simulink model "AL1adaptive"  (R2022b)
settings: Solver=ode45  StartTime=0.0  StopTime=10  RelTol=1e-6  EnableMultiTasking=on
values from neighbouring files (symbols this model uses):
  Am = (A-B*K1)    [AL1initialize.m]
  Bm = B    [AL1initialize.m]
  Bum = [     1     0     0     0     0     0     0     0;     0     1     0     0     0     0     0     0;     0     0     0     0     0     0     0     0;     0     0     0     0     0     0     0     0;     0     0     0     0     0     0     0     0;     0     0     0     0     0     0     0     0;     0     0     1     0     0     0     0     0;     0     0     0     1     0     0     0     0;     0  ...(+189 chars)    [AL1initialize.m]
  C_full = [     0 0 0     0 0 0    1 0 0    0 0 0;     0 0 0     0 0 0    0 1 0    0 0 0;     0 0 0     0 0 0    0 0 1    0 0 0;     0 0 0     0 0 0    0 0 0    1 0 0;     0 0 0     0 0 0    0 0 0    0 1 0;     0 0 0     0 0 0    0 0 0    0 0 1]    [AL1initialize.m]
  D = zeros(4,4)    [AL1initialize.m]
  Deltabound = 1    [AL1initialize.m]
  HD = ss(zeros(4,4),eye(4),eye(4),zeros(4,4))    [AL1initialize.m]
  HmHum = ss(HmHumprop)    [AL1initialize.m]
  K1 = lqr(A,B,Q,R)    [AL1initialize.m]
  K2 = eye(4)*10    [AL1initialize.m]
  Kg = -(C*Am^-1*Bm)^-1    [AL1initialize.m]
  Lambda = [ ... (first row only)    [AL1initialize.m]
  PBmG = P*Bm*Gamma    [AL1initialize.m]
  PBumG = P*Bum*Gamma    [AL1initialize.m]
  V_trim = [v_trim; v_trim; v_trim; v_trim]    [AL1initialize.m]
  vfail = (12)^(1/3.88)    (= 1.89731524545)    [AL1initialize.m]
  Vmax = 12.5    [AL1initialize.m]
  x_initial = [0;0;0;0;0;0;0;0;0;0;0;0]    [AL1initialize.m]
libraries: Projection x8, matrix_library x6, simulink_extras x4
settings Model: Creator=oldmao  LastModifiedBy=HY
settings SolverCC: AlgebraicLoopSolver=TrustRegion
settings DataIOCC: LimitDataPoints=on  SaveFormat=Array  SignalLoggingSaveFormat=ModelDataLogs  ReturnWorkspaceOutputs=off
settings OptimizationCC: ExpressionDepthLimit=2147483647  LifeSpan=inf
settings DebuggingCC: UnderspecifiedInitializationDetection=Classic  MergeDetectMultiDrivingBlocksExec=none  SolverPrmCheckMsg=warning  FcnCallInpInsideContextMsg=warning  UnconnectedInputMsg=warning  UnconnectedOutputMsg=warning  UnconnectedLineMsg=warning  AllowSymbolicDim=off  StateNameClashWarn=warning  SFUnexpectedBacktrackingDiag=warning  SFNoUnconditionalDefaultTransitionDiag=warning  SFExecutionAtInitializationDiag=none  SFMachineParentedDataDiag=warning  ArithmeticOperatorsInVariantConditions=warning
settings HardwareCC: ProdBitPerPointer=32  ProdBitPerSizeT=32  ProdBitPerPtrDiffT=32  ProdLargestAtomicFloat=None  ProdIntDivRoundTo=Undefined  ProdEndianess=Unspecified  ProdWordSize=32  ProdHWDeviceType=32-bit Generic
settings ModelReferenceCC: EnableRefExpFcnMdlSchedulingChecks=on  PropagateSignalLabelsOutOfModel=off
settings SFSimCC: SimUseLocalCustomCode=off  CustomCodeUndefinedFunction=UseInterfaceOnly
settings RTWCC: RTWUseLocalCustomCode=off
settings CodeAppCC: StateflowObjectComments=on
settings GRTTargetCC: TargetLangStandard=C89/C90 (ANSI)  CombineOutputUpdateFcns=off  GRTInterface=on
settings ConfigComp: CovMetricSettings=dw  CovSaveCumulativeToWorkspaceVar=on  CovSaveSingleToWorkspaceVar=on  CovExternalEMLEnable=off  CovSFcnEnable=off

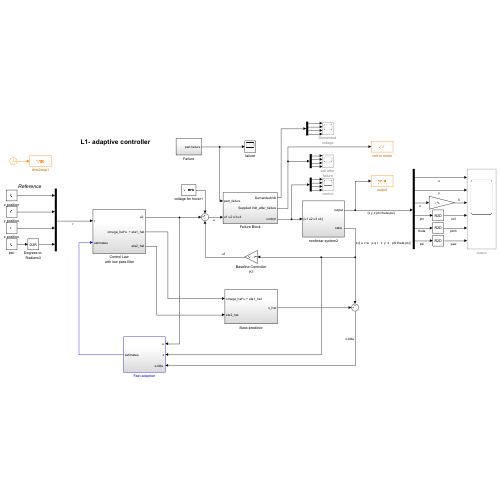
[thumbnail: Simulink's stored preview of the top-level diagram]
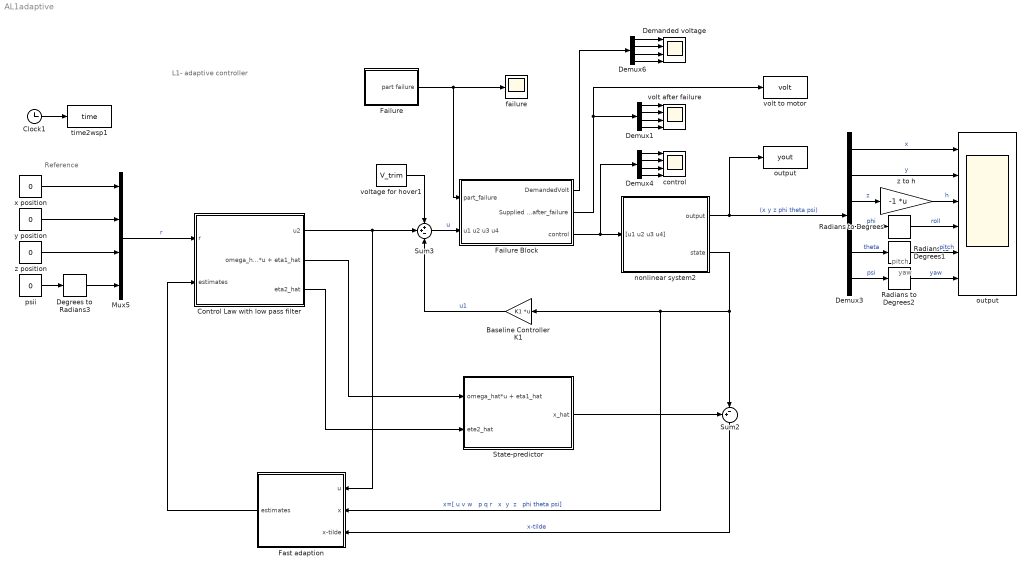
== system AL1adaptive ==
  note: Reference
  note: yaw
  note: pitch
  note: L1- adaptive controller
  Baseline Controller K1 : Gain  Gain=K1  Multiplication=Matrix(K*u) (u vector)
  Clock1 : Clock
  Control Law with low pass filter : Subsystem
  Degrees to Radians3 : simulink_extras/Transformations/Degrees to Radians
  Demanded voltage : Scope  NumInputPorts=4
  Demux1 : Demux
  Demux3 : Demux  Outputs=6
  Demux4 : Demux
  Demux6 : Demux
  Failure : Subsystem
  Failure Block : Subsystem
  Fast adaption : Subsystem
  Mux5 : Mux
  Radians to Degrees : simulink_extras/Transformations/Radians to Degrees
  Radians to Degrees1 : simulink_extras/Transformations/Radians to Degrees
  Radians to Degrees2 : simulink_extras/Transformations/Radians to Degrees
  State-predictor : Subsystem
  Sum2 : Sum  Inputs=+-|
  Sum3 : Sum  Inputs=++-
  "control " : Scope  NumInputPorts=4
  failure : Scope
  nonlinear system2 : Subsystem
  output : ToWorkspace  VariableName=yout  SaveFormat=Structure With Time  SampleTime=-1
  "output " : Scope  NumInputPorts=6
  "psii " : Constant  Value=0
  time2wsp1 : ToWorkspace  VariableName=time  SampleTime=-1
  volt after failure : Scope  NumInputPorts=4
  volt to motor : ToWorkspace  VariableName=volt  SaveFormat=Structure With Time  SampleTime=-1
  voltage for hover1 : Constant  Value=V_trim
  x position : Constant  Value=0
  "y position " : Constant  Value=0
  z position : Constant  Value=0
  z to h : Gain  Gain=-1  Multiplication=Matrix(K*u)
  wires:
  Clock1/1 -> time2wsp1/1
  Sum2/1 -> Fast adaption/3("x-tilde ")  "x-tilde"
  Sum3/1 -> Failure Block/2(u1 u2 u3 u4)  "u"
  Demux3/3 -> z to h/1  "z"
  Baseline Controller K1/1 -> Sum3/3  "u1"
  Failure Block/3(control) -> Demux4/1, nonlinear system2/1("[u1 u2 u3 u4]")
  Demux1/1 -> volt after failure/1
  Demux1/3 -> volt after failure/3
  Demux1/2 -> volt after failure/2
  Demux1/4 -> volt after failure/4
  Demux4/1 -> "control "/1
  Demux4/3 -> "control "/3
  Demux4/2 -> "control "/2
  Demux4/4 -> "control "/4
  Demux3/4 -> Radians to Degrees/1  "phi"
  Demux3/5 -> Radians to Degrees1/1  "theta"
  Demux3/6 -> Radians to Degrees2/1  "psi"
  Demux3/1 -> "output "/1  "x"
  nonlinear system2/2("state ") -> Baseline Controller K1/1, Fast adaption/2(x), Sum2/2  "x=[ u v w   p q r   x  y  z   phi theta psi]"
  "psii "/1 -> Degrees to Radians3/1
  z position/1 -> Mux5/3
  "y position "/1 -> Mux5/2
  x position/1 -> Mux5/1
  voltage for hover1/1 -> Sum3/1
  nonlinear system2/1(output) -> Demux3/1, output/1  "(x y z phi theta psi)"
  Radians to Degrees2/1 -> "output "/6  "yaw"
  Radians to Degrees1/1 -> "output "/5  "pitch"
  Radians to Degrees/1 -> "output "/4  "roll"
  z to h/1 -> "output "/3  "h"
  Demux3/2 -> "output "/2  "y"
  Failure/1(part failure) -> Failure Block/1("part_failure "), failure/1
  Demux6/1 -> Demanded voltage/1
  Demux6/3 -> Demanded voltage/3
  Demux6/2 -> Demanded voltage/2
  Demux6/4 -> Demanded voltage/4
  Failure Block/1(" DemandedVolt") -> Demux6/1
  Failure Block/2(Supplied Volt_after_failure) -> volt to motor/1, Demux1/1
  Degrees to Radians3/1 -> Mux5/4
  State-predictor/1(x_hat) -> Sum2/1
  Control Law with low pass filter/1("u2 ") -> Fast adaption/1(u), Sum3/2
  Mux5/1 -> Control Law with low pass filter/1(r)  "r"
  Fast adaption/1(estimates) -> Control Law with low pass filter/2(estimates)
  Control Law with low pass filter/2(omega_hat*u + eta1_hat) -> State-predictor/1(omega_hat*u + eta1_hat)
  Control Law with low pass filter/3(eta2_hat) -> State-predictor/2(ete2_hat)

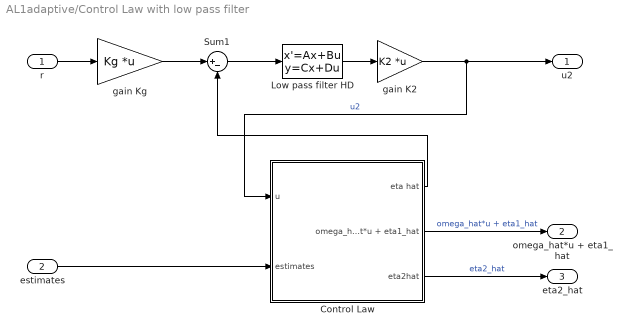
== system AL1adaptive/Control Law with low pass filter ==
  r : Inport
  estimates : Inport  Port=2
  Control Law : Subsystem
  Low pass filter HD : StateSpace  A=HD.a  B=HD.b  C=HD.c  D=HD.d  InitialCondition=0
  Sum1 : Sum  Inputs=|+-
  gain K2 : Gain  Gain=K2  Multiplication=Matrix(K*u) (u vector)
  gain Kg : Gain  Gain=Kg  Multiplication=Matrix(K*u)
  "u2 " : Outport
  omega_hat*u + eta1_hat : Outport  Port=2
  eta2_hat : Outport  Port=3
  wires:
  estimates/1 -> Control Law/2(estimates)
  Low pass filter HD/1 -> gain K2/1
  r/1 -> gain Kg/1
  Control Law/1(eta hat) -> Sum1/2
  gain K2/1 -> Control Law/1(u), "u2 "/1  "u2"
  Sum1/1 -> Low pass filter HD/1
  gain Kg/1 -> Sum1/1
  Control Law/2(omega_hat*u + eta1_hat) -> omega_hat*u + eta1_hat/1  "omega_hat*u + eta1_hat"
  Control Law/3(eta2hat) -> eta2_hat/1  "eta2_hat"

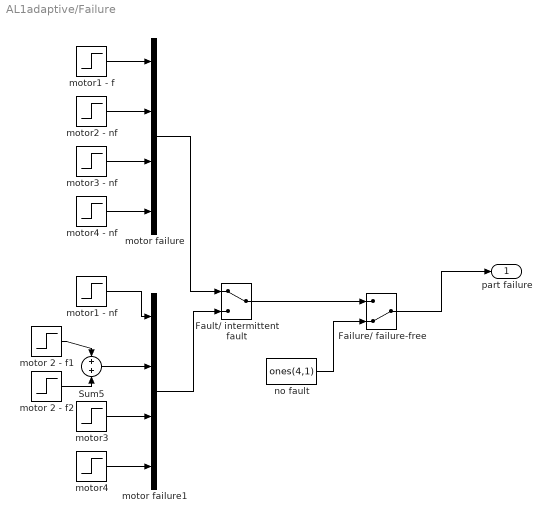
== system AL1adaptive/Failure ==
  Failure/ failure-free : ManualSwitch  CurrentSetting=0
  Fault/ intermittent fault : ManualSwitch
  Sum5 : Sum  Inputs=+|+
  motor 2 - f1 : Step  Before=1  After=0.5  SampleTime=0
  motor 2 - f2 : Step  Time=3  After=0.5  SampleTime=0
  motor failure : Concatenate  NumInputs=4
  motor failure1 : Concatenate  NumInputs=4
  motor1 - f : Step  Before=1  After=(vfail)^(3.88)  SampleTime=0
  motor1 - nf : Step  Time=5  Before=1  SampleTime=0
  motor2 - nf : Step  Before=1  SampleTime=0
  motor3 : Step  Time=5  Before=1  SampleTime=0
  motor3 - nf : Step  Time=5  Before=1  SampleTime=0
  motor4 : Step  Time=5  Before=1  SampleTime=0
  motor4 - nf : Step  Time=5  Before=1  SampleTime=0
  no fault : Constant  Value=ones(4,1)
  part failure : Outport
  wires:
  motor4/1 -> motor failure1/4
  motor3/1 -> motor failure1/3
  motor failure1/1 -> Fault/ intermittent fault/2
  motor 2 - f2/1 -> Sum5/2
  motor 2 - f1/1 -> Sum5/1
  motor4 - nf/1 -> motor failure/4
  motor3 - nf/1 -> motor failure/3
  motor2 - nf/1 -> motor failure/2
  motor1 - f/1 -> motor failure/1
  motor failure/1 -> Fault/ intermittent fault/1
  Fault/ intermittent fault/1 -> Failure/ failure-free/1
  Failure/ failure-free/1 -> part failure/1
  no fault/1 -> Failure/ failure-free/2
  motor1 - nf/1 -> motor failure1/1
  Sum5/1 -> motor failure1/2

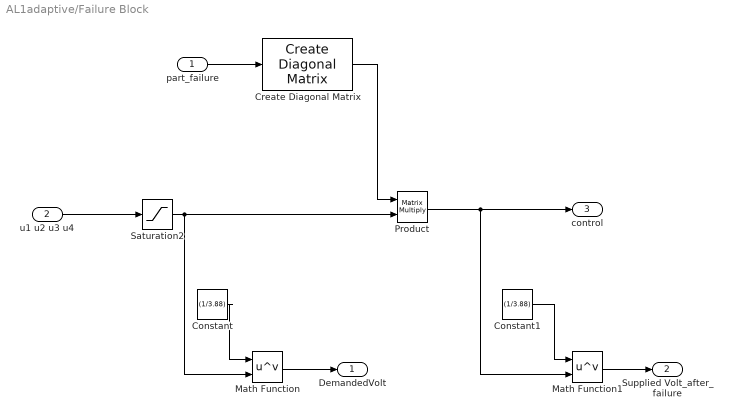
== system AL1adaptive/Failure Block ==
  "part_failure " : Inport
  u1 u2 u3 u4 : Inport  Port=2
  Constant : Constant  Value=(1/3.88)
  Constant1 : Constant  Value=(1/3.88)
  Create Diagonal Matrix : matrix_library/Create Diagonal Matrix
  Math Function : Math  Operator=pow
  Math Function1 : Math  Operator=pow
  Product : Product  Multiplication=Matrix(*)  RndMeth=Zero
  Saturation2 : Saturate  UpperLimit=Vmax^(3.88)  LowerLimit=0
  " DemandedVolt" : Outport
  Supplied Volt_after_failure : Outport  Port=2
  control : Outport  Port=3
  wires:
  Create Diagonal Matrix/1 -> Product/1
  "part_failure "/1 -> Create Diagonal Matrix/1
  Math Function/1 -> " DemandedVolt"/1
  u1 u2 u3 u4/1 -> Saturation2/1
  Saturation2/1 -> Product/2, Math Function/2
  Product/1 -> Math Function1/2, control/1
  Constant/1 -> Math Function/1
  Constant1/1 -> Math Function1/1
  Math Function1/1 -> Supplied Volt_after_failure/1

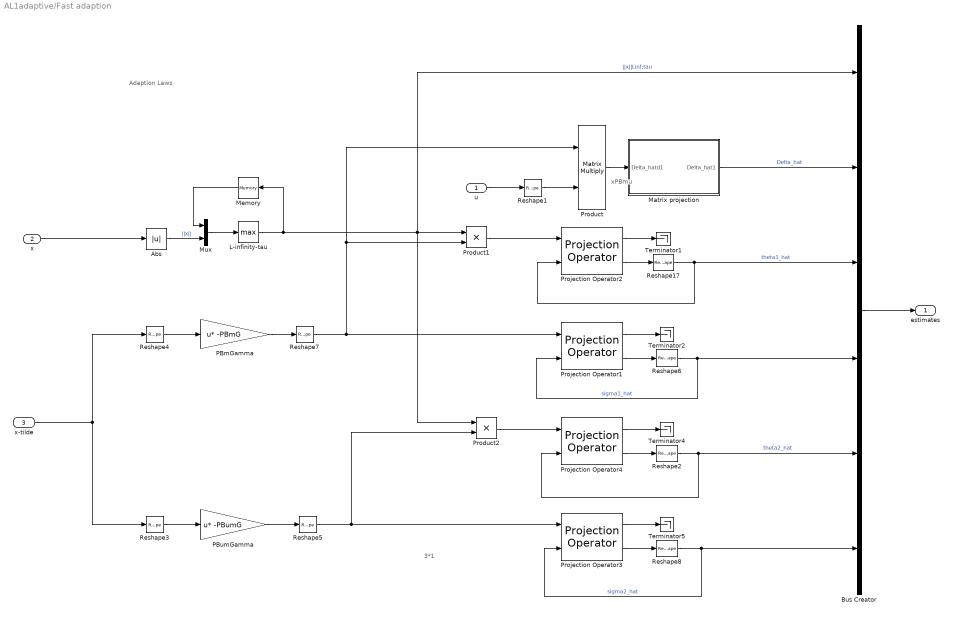
== system AL1adaptive/Fast adaption ==
  note: Adaption Laws
  note: xPBmu
  note: 3*1
  u : Inport
  x : Inport  Port=2
  "x-tilde " : Inport  Port=3
  Abs : Abs  SaturateOnIntegerOverflow=off
  Bus Creator : BusCreator  Inputs=6
  L-infinity-tau : MinMax  Function=max
  Matrix projection : Subsystem
  Memory : Memory
  Mux : Mux  Inputs=2
  PBmGamma : Gain  Gain=-PBmG  Multiplication=Matrix(u*K)
  PBumGamma : Gain  Gain=-PBumG  Multiplication=Matrix(u*K)
  Product : Product  Multiplication=Matrix(*)  RndMeth=Zero
  Product1 : Product  RndMeth=Zero
  Product2 : Product  RndMeth=Zero
  Projection Operator1 : Projection/Projection Operator  EpsilonTheta=.1  Prmax=sigama1hatbound  Prcenter=0  Pr0=0
  Projection Operator2 : Projection/Projection Operator  EpsilonTheta=.1  Prmax=theta1hatbound  Prcenter=0  Pr0=0
  Projection Operator3 : Projection/Projection Operator  EpsilonTheta=.1  Prmax=sigama2hatbound  Prcenter=0  Pr0=0
  Projection Operator4 : Projection/Projection Operator  EpsilonTheta=.1  Prmax=theta2hatbound  Prcenter=0  Pr0=0
  Reshape1 : Reshape  OutputDimensionality=Row vector (2-D)
  Reshape{2,5..8,17} (6 alike) : Reshape  OutputDimensionality=Column vector (2-D)
  Reshape3 : Reshape  OutputDimensionality=Row vector (2-D)
  Reshape4 : Reshape  OutputDimensionality=Row vector (2-D)
  Terminator{1..2,4..5} (4 alike) : Terminator
  estimates : Outport
  wires:
  x/1 -> Abs/1
  Projection Operator2/2 -> Reshape17/1
  Projection Operator2/1 -> Terminator1/1
  Reshape17/1 -> Projection Operator2/2, Bus Creator/3  "theta1_hat"
  Projection Operator1/2 -> Reshape6/1
  Projection Operator1/1 -> Terminator2/1
  u/1 -> Reshape1/1
  Reshape4/1 -> PBmGamma/1
  Reshape1/1 -> Product/2
  Product1/1 -> Projection Operator2/1
  PBmGamma/1 -> Reshape7/1
  "x-tilde "/1 -> Reshape4/1, Reshape3/1
  Reshape7/1 -> Projection Operator1/1, Product1/2, Product/1
  Projection Operator4/2 -> Reshape2/1
  Projection Operator4/1 -> Terminator4/1
  Projection Operator3/2 -> Reshape8/1
  Projection Operator3/1 -> Terminator5/1
  Reshape3/1 -> PBumGamma/1
  Product2/1 -> Projection Operator4/1
  PBumGamma/1 -> Reshape5/1
  Reshape5/1 -> Product2/2, Projection Operator3/1
  Reshape6/1 -> Projection Operator1/2, Bus Creator/4  "sigma1_hat"
  Product/1 -> Matrix projection/1(Delta_hatd1)
  Matrix projection/1(Delta_hat1) -> Bus Creator/2  "Delta_hat"
  Reshape2/1 -> Projection Operator4/2, Bus Creator/5  "theta2_hat"
  Reshape8/1 -> Projection Operator3/2, Bus Creator/6  "sigma2_hat"
  Abs/1 -> Mux/2  "||x||"
  Mux/1 -> L-infinity-tau/1
  Memory/1 -> Mux/1
  L-infinity-tau/1 -> Memory/1, Product2/1, Bus Creator/1, Product1/1  "||x||Linf;tau"
  Bus Creator/1 -> estimates/1

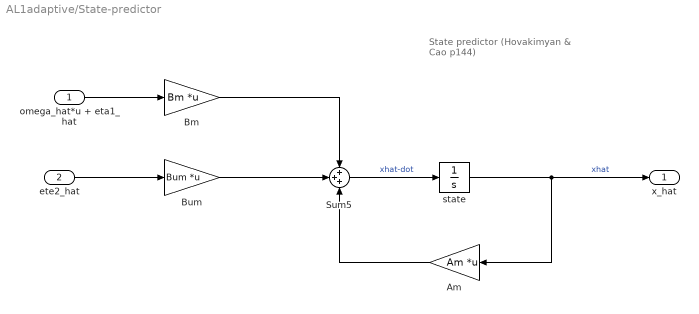
== system AL1adaptive/State-predictor ==
  note: State predictor
      | (Hovakimyan & Cao p144)
  omega_hat*u + eta1_hat : Inport
  ete2_hat : Inport  Port=2
  Am : Gain  Gain=Am  Multiplication=Matrix(K*u) (u vector)
  Bm : Gain  Gain=Bm  Multiplication=Matrix(K*u) (u vector)
  Bum : Gain  Gain=Bum  Multiplication=Matrix(K*u) (u vector)
  Sum5 : Sum  Inputs=+++
  state : Integrator  InitialCondition=x_initial
  x_hat : Outport
  wires:
  Am/1 -> Sum5/3
  Sum5/1 -> state/1  "xhat-dot"
  state/1 -> x_hat/1, Am/1  "xhat"
  ete2_hat/1 -> Bum/1
  omega_hat*u + eta1_hat/1 -> Bm/1
  Bum/1 -> Sum5/2
  Bm/1 -> Sum5/1

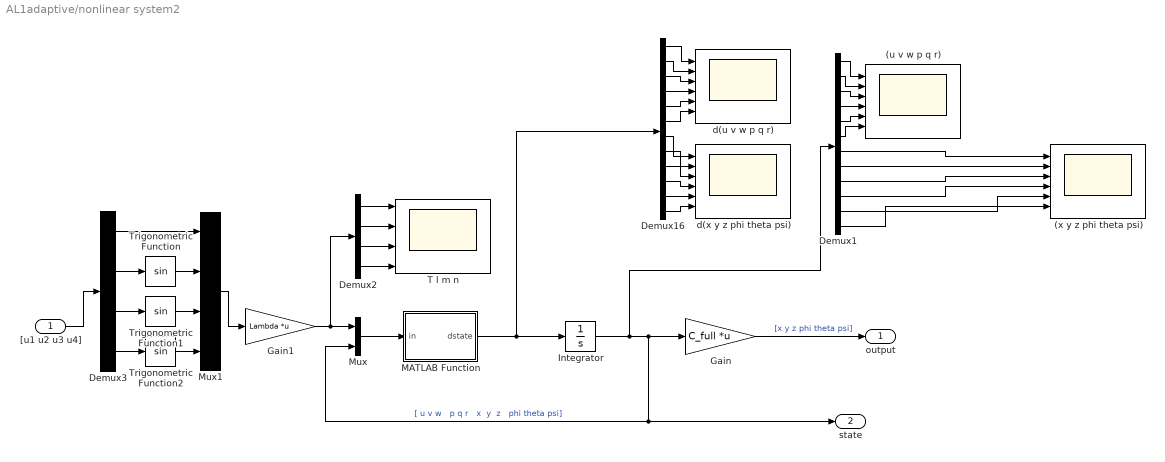
== system AL1adaptive/nonlinear system2 ==
  "[u1 u2 u3 u4]" : Inport
  (u v w p q r) : Scope  NumInputPorts=6
  (x y z phi theta psi) : Scope  NumInputPorts=6
  Demux1 : Demux  Outputs=12
  Demux16 : Demux  Outputs=12
  Demux2 : Demux
  Demux3 : Demux
  Gain : Gain  Gain=C_full  Multiplication=Matrix(K*u)
  Gain1 : Gain  Gain=Lambda  Multiplication=Matrix(K*u)
  Integrator : Integrator  InitialCondition=x_initial
  MATLAB Function : MATLAB Function  TreatAsAtomicUnit=on
  Mux : Mux  Inputs=2
  Mux1 : Mux
  T l m n : Scope  NumInputPorts=4
  Trigonometric Function : Trigonometry
  Trigonometric Function1 : Trigonometry
  Trigonometric Function2 : Trigonometry
  d(u v w p q r) : Scope  NumInputPorts=6
  d(x y z phi theta psi) : Scope  NumInputPorts=6
  output : Outport
  "state " : Outport  Port=2
  wires:
  Gain/1 -> output/1  "[x y z phi theta psi]"
  Mux/1 -> MATLAB Function/1(in)
  Integrator/1 -> Demux1/1, Gain/1, "state "/1, Mux/2  "[ u v w   p q r   x  y  z   phi theta psi]"
  Demux16/1 -> d(u v w p q r)/1
  Demux16/3 -> d(u v w p q r)/3
  Demux16/2 -> d(u v w p q r)/2
  Demux16/4 -> d(u v w p q r)/4
  Demux16/12 -> d(x y z phi theta psi)/6
  Demux16/11 -> d(x y z phi theta psi)/5
  Demux16/10 -> d(x y z phi theta psi)/4
  Demux16/9 -> d(x y z phi theta psi)/3
  Demux16/8 -> d(x y z phi theta psi)/2
  Demux16/7 -> d(x y z phi theta psi)/1
  Demux16/5 -> d(u v w p q r)/5
  Demux16/6 -> d(u v w p q r)/6
  Demux1/1 -> (u v w p q r)/1
  Demux1/3 -> (u v w p q r)/3
  Demux1/2 -> (u v w p q r)/2
  Demux1/4 -> (u v w p q r)/4
  Demux1/12 -> (x y z phi theta psi)/6
  Demux1/11 -> (x y z phi theta psi)/5
  Demux1/10 -> (x y z phi theta psi)/4
  Demux1/9 -> (x y z phi theta psi)/3
  Demux1/8 -> (x y z phi theta psi)/2
  Demux1/7 -> (x y z phi theta psi)/1
  Demux1/5 -> (u v w p q r)/5
  Demux1/6 -> (u v w p q r)/6
  Gain1/1 -> Demux2/1, Mux/1
  MATLAB Function/1(dstate) -> Demux16/1, Integrator/1
  Demux2/1 -> T l m n/1
  Demux2/2 -> T l m n/2
  Demux2/3 -> T l m n/3
  Demux2/4 -> T l m n/4
  Demux3/3 -> Trigonometric Function1/1
  Demux3/2 -> Trigonometric Function/1
  Demux3/1 -> Mux1/1
  Demux3/4 -> Trigonometric Function2/1
  "[u1 u2 u3 u4]"/1 -> Demux3/1
  Trigonometric Function1/1 -> Mux1/3
  Trigonometric Function/1 -> Mux1/2
  Trigonometric Function2/1 -> Mux1/4
  Mux1/1 -> Gain1/1

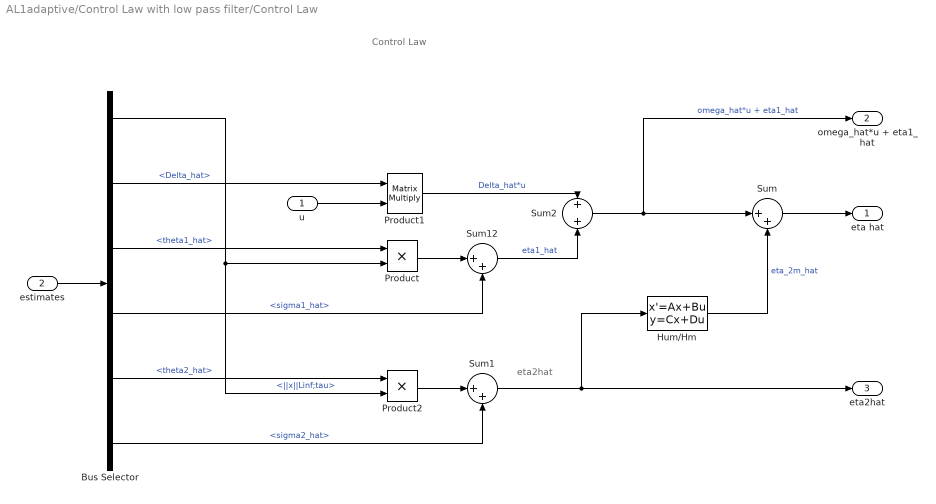
== system AL1adaptive/Control Law with low pass filter/Control Law ==
  note: Control Law
  note: eta2hat
  u : Inport
  estimates : Inport  Port=2
  Bus Selector : BusSelector  OutputSignals=||x||Linf;tau,Delta_hat,theta1_hat,sigma1_hat,theta2_hat,sigma2_hat
  "Hum/Hm " : StateSpace  A=HmHum.a  B=HmHum.b  C=HmHum.c  D=HmHum.d  InitialCondition=0
  Product : Product  RndMeth=Zero
  Product1 : Product  Multiplication=Matrix(*)  RndMeth=Zero
  Product2 : Product  RndMeth=Zero
  Sum : Sum  Inputs=|++
  Sum1 : Sum  Inputs=|++
  Sum12 : Sum  Inputs=|++
  Sum2 : Sum  Inputs=+|+
  eta hat : Outport
  omega_hat*u + eta1_hat : Outport  Port=2
  eta2hat : Outport  Port=3
  wires:
  Bus Selector/3 -> Product/1  "<theta1_hat>"
  Bus Selector/4 -> Sum12/2  "<sigma1_hat>"
  Bus Selector/5 -> Product2/1  "<theta2_hat>"
  Product2/1 -> Sum1/1
  Bus Selector/6 -> Sum1/2  "<sigma2_hat>"
  Bus Selector/2 -> Product1/1  "<Delta_hat>"
  u/1 -> Product1/2
  Sum1/1 -> "Hum/Hm "/1, eta2hat/1
  Sum/1 -> eta hat/1
  "Hum/Hm "/1 -> Sum/2  "eta_2m_hat"
  Product/1 -> Sum12/1
  Sum2/1 -> omega_hat*u + eta1_hat/1, Sum/1  "omega_hat*u + eta1_hat"
  Sum12/1 -> Sum2/2  "eta1_hat"
  Product1/1 -> Sum2/1  "Delta_hat*u"
  Bus Selector/1 -> Product2/2, Product/2  "<||x||Linf;tau>"
  estimates/1 -> Bus Selector/1

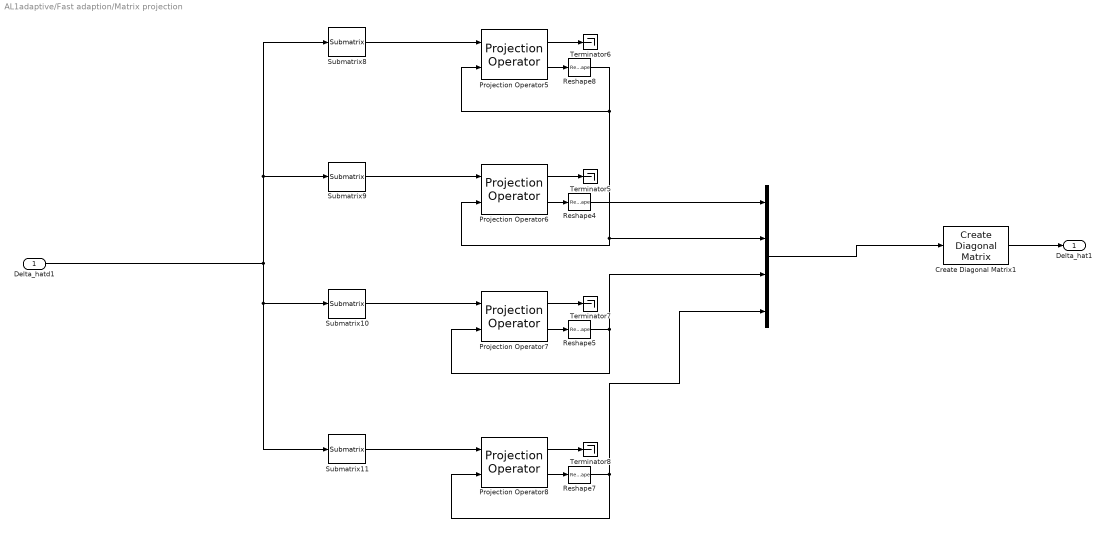
== system AL1adaptive/Fast adaption/Matrix projection ==
  Delta_hatd1 : Inport
  " " : Concatenate  NumInputs=4
  Create Diagonal Matrix1 : matrix_library/Create Diagonal Matrix
  Projection Operator5 : Projection/Projection Operator  EpsilonTheta=.1  Prmax=Deltabound/2  Prcenter=0.5  Pr0=1
  Projection Operator6 : Projection/Projection Operator  EpsilonTheta=.1  Prmax=Deltabound/2  Prcenter=0.5  Pr0=1
  Projection Operator7 : Projection/Projection Operator  EpsilonTheta=.1  Prmax=Deltabound/2  Prcenter=0.5  Pr0=1
  Projection Operator8 : Projection/Projection Operator  EpsilonTheta=0.1  Prmax=Deltabound/2  Prcenter=0.5  Pr0=1
  Reshape{4..5,7..8} (4 alike) : Reshape  OutputDimensionality=Column vector (2-D)
  Submatrix10 : matrix_library/Submatrix  RowSpan=One row  RowStartMode=Index  RowStartIndex=3  RowEndMode=Last  RowEndIndex=1  ColSpan=One column  ColStartMode=Index  ColStartIndex=3  ColEndMode=Last  ColEndIndex=1
  Submatrix11 : matrix_library/Submatrix  RowSpan=One row  RowStartMode=Index  RowStartIndex=4  RowEndMode=Last  RowEndIndex=1  ColSpan=One column  ColStartMode=Index  ColStartIndex=4  ColEndMode=Last  ColEndIndex=1
  Submatrix8 : matrix_library/Submatrix  RowSpan=One row  RowStartMode=Index  RowStartIndex=1  RowEndMode=Last  RowEndIndex=1  ColSpan=One column  ColStartMode=Index  ColStartIndex=1  ColEndMode=Last  ColEndIndex=1
  Submatrix9 : matrix_library/Submatrix  RowSpan=One row  RowStartMode=Index  RowStartIndex=2  RowEndMode=Last  RowEndIndex=1  ColSpan=One column  ColStartMode=Index  ColStartIndex=2  ColEndMode=Last  ColEndIndex=1
  Terminator{5..8} (4 alike) : Terminator
  Delta_hat1 : Outport
  wires:
  Submatrix8/1 -> Projection Operator5/1
  Projection Operator5/1 -> Terminator6/1
  Projection Operator5/2 -> Reshape8/1
  Submatrix10/1 -> Projection Operator7/1
  Projection Operator7/1 -> Terminator7/1
  Projection Operator7/2 -> Reshape5/1
  Reshape5/1 -> " "/3, Projection Operator7/2
  Reshape4/1 -> Projection Operator6/2, " "/2
  Projection Operator6/1 -> Terminator5/1
  Projection Operator6/2 -> Reshape4/1
  Create Diagonal Matrix1/1 -> Delta_hat1/1
  Submatrix9/1 -> Projection Operator6/1
  Reshape8/1 -> " "/1, Projection Operator5/2
  Submatrix11/1 -> Projection Operator8/1
  Projection Operator8/1 -> Terminator8/1
  Projection Operator8/2 -> Reshape7/1
  Reshape7/1 -> " "/4, Projection Operator8/2
  Delta_hatd1/1 -> Submatrix11/1, Submatrix10/1, Submatrix8/1, Submatrix9/1
  " "/1 -> Create Diagonal Matrix1/1

== matlab function AL1adaptive/nonlinear system2/MATLAB Function ==
  data: in input; dstate output
function dstate = Eom(in)
%#codegen
%Function used for simulating the quadrotor dynamics and outputs its current state space vector.
%And this function is called during the Simulink simulation by a interpreted Matlab function.
%% Input force and moments
T=in(1);
L=in(2);
M=in(3);
N=in(4);
%% System state
u=in(5);
v=in(6);
w=in(7);
p=in(8);
q=in(9);
r=in(10);
%x=in(11);
%y=in(12);
%z=in(13);
phi=in(14);
theta=in(15);
psi=in(16);
%% Define constants and Rotaion maxtrix
I=[1.224 0 0;...
 0 6.688 0;...
 0 0 6.688];% Principal moment of inertia matrix
m=24.55; %quadrotor mass
g=9.81;
%rotating about x axies
% Rx=[1 0 0;...
%         0 cos(phi) sin(phi);...
%         0 -sin(phi) cos(phi)];
% %rotating about y
% Ry=[cos(theta) 0 -sin(theta);...
%         0 1 0
%         sin(theta) 0 cos(theta)];
% %rotating about z
% Rz=[cos(psi) sin(psi) 0;...
%         -sin(psi) cos(psi) 0;...
%         0 0 1];
%  %quadrotor Rzxy: from earth to body axies
% Rzxy=Rz*Rx*Ry;  
% Rxyz=Rx*Ry*Rz;
% %Tranfermation matrix for body rate to euler rate:
% Jxyz=[1     tan(theta)*sin(phi)     tan(theta)*cos(phi) ;...
%       0        cos(phi)            -sin(phi) ;...
%       0        sin(phi)/cos(theta)  cos(phi)/cos(theta)];
%  
% 
% Jzxy=[          cos(psi)         -sin(psi) 0;...
%  sin(psi)/cos(phi)  cos(psi)/cos(phi)  0;...
%  sin(psi)*tan(phi)  cos(psi)*tan(phi)  1];
% %% Equation of Motion
% xdydzd=transpose(Rxyz)*[u;v;w];
% udvdwd=-1/m*[0;0;T]+Rxyz*[0;0;g]-cross([p;q;r],[u;v;w]);
% pdqdrd=I^-1*([L;M;N]-cross([p;q;r],I*[p;q;r]));
% phidthetadpsid=Jxyz*[p;q;r];
% %% state derivatives
% dstate=[udvdwd;pdqdrd;xdydzd;phidthetadpsid];

dstate=[-g*sin(theta) - (q*w-r*v); % u
  g*cos(theta)*sin(phi)- (r*u - p*w); % v
 -T/m + g*cos(theta)*cos(phi)- (p*v-q*u);% w
 L/I(1,1)-(I(3,3) - I(2,2))*q*r/I(1,1); % p
 M/I(2,2)-(I(1,1) - I(3,3))*r*p/I(2,2); % q
 N/I(3,3)-(I(2,2) - I(1,1))*p*q/I(3,3); % r
 cos(psi)*cos(theta)*u + (cos(psi)*sin(theta)*sin(phi)-sin(psi)*cos(phi))*v + (cos(psi)*sin(theta)*cos(phi)+sin(psi)*sin(phi))*w; %x
 sin(psi)*cos(theta)*u + (sin(psi)*sin(theta)*sin(phi)+cos(psi)*cos(phi))*v + (sin(psi)*sin(theta)*cos(phi)-cos(psi)*sin(phi))*w; %y 
-sin(theta)*u + cos(theta)*sin(phi)*v + cos(theta)*cos(phi)*w; %z
p + tan(theta)*sin(phi)*q + tan(theta)*cos(phi)*r; %phi
cos(phi)*q - sin(phi)*r; %theta
sin(phi)*q/cos(theta) +  cos(phi)*r/cos(theta) ]; % psi
end
